simulink model "mfordmodel_v1"  (R2023a)
settings: Solver=ode45  StartTime=0.0  StopTime=10.0  RelTol=1e-3  EnableMultiTasking=on
undefined symbols (not defined in the file): ABV_RATIO_SW, AC_OFF_DLY, ACLOD, AUTO_TRNS_SW, BRAKE_DNDT_X, BZZRPM, BZZRPM_ALT, BZZTM, BZZTM_ALT, CMD_LITOFF, CMD_STABLE, CO_ST_ECT__A, COOL_BASE, DAS_BKDLY_A, DAS_CNT, DAS_CTDLY, DAS_LC_SW__A, DASCLP_5INH, DASCTL, DASMHYST, DASMPH, DEBYCP, DES_BASE, DPNEU_MUL, DSDRPM_DN_TC, DSDRPM_OFF, DSDRPM_UP_TC, EDF_DELAY, EDFHP, ETC_CL_TP, ETC_HP, GR_CM_CREEP, HCAM_ACT_CLP, HEDFHP, HEDFRPM, HICAM_PS, IAC_CAL_SW, IAC_ER_TM1, IAC_ER_TM2, IAC_ER_TM4, IAC_HI_LIM__A, IAC_ISFL_OBD, IAC_KAM_SW, IAC_LO_LIM__A, IAC_MON_TM, IAC_OT_REQ, IAC_RUN_TM, IAC_TP_OBD, IAC_TR_DAS, IAC_TST_DC, ID_DAS__A, ID_NOVS__A, IDVS_CH__A, IDVS_SL__A, IPSI_SW, IPSIDLY, IS_DRBASE__A, IS_DRBASE_A__A, IS_NUBASE__A, IS_NUBASE_A__A ... (+35)
libraries: simulink x2
(part 12 of 12)

== stateflow chart mfordmodel_v1/iac_v04_001_001/normal_mode/iscflg_module/idle_drive_rpm_controller/idle_drive_rpm_controller_ctl ==
  state idle_drive_rpm_init [parallel]
    settings: executionOrder=1
    idle_drive_rpm_init -> (junction 13) : trig
    (default) -> (junction 13) : trig
    (junction 13) -> (junction 14) : {
        | ml_init_sw = 2;
        | ml_idnerr_sw = 1;
        | do_idnerr_fil_calc;
        | do_idle_ppm_calc;
        | }
  state idle_drive_rpm_control [parallel]
    settings: executionOrder=2
    idle_drive_rpm_control -> (junction 15) : trig_idle_drive_rpm_controller
    (default) -> (junction 15) : trig_idle_drive_rpm_controller
    (junction 15) -> (junction 18) [order 2] : /* idle_drive_rpm_controller_initialisation() */
        | {
        | idle_drive_rpm_init.trig;
        | }
    (junction 15) -> (junction 16) [order 1] : [ ml_idrv_init_flg == 0 ]
        | {
        | ml_init_sw = 1;
        | do_idnerr_fil_calc;
        | }
    (junction 16) -> (junction 17) [order 2] : {
        | ml_idnerr_sw = 2;
        | }
    (junction 16) -> (junction 17) [order 1] : [ fabs(idnerr_fil) >= ID_DB_CAL ]
        | {
        | ml_idnerr_sw = 1;
        | }
    (junction 17) -> (junction 18) : {
        | do_idle_ppm_calc;
        | }
  data: ml_init_sw output uint8 size=1; ml_idrv_init_flg input boolean size=1; idnerr_fil input double size=1; ID_DB_CAL parameter double size=1; idnerr__A input double size=1; ml_idnerr_sw output int8 size=1
  events: trig local EITHER_EDGE_EVENT; trig_idle_drive_rpm_controller input FUNCTION_CALL_EVENT; do_idle_ppm_calc output FUNCTION_CALL_EVENT; do_idnerr_fil_calc output FUNCTION_CALL_EVENT

== stateflow chart mfordmodel_v1/iac_v04_001_001/normal_mode/activate_kam/activate_kam_ctl ==
  state isflag_update [parallel]
    settings: executionOrder=1
    isflag_update -> (junction 50) : trig   /* Determine which cell in 'isckam[]'
        |            will be used for learning: isflag =
        |            0 = No A/C request, neutral.
        |            1 = A/C request, neutral.
        |            2 = No A/C request, drive.
        |            3 = A/C request, drive.  */
    (default) -> (junction 50) : trig
    (junction 50) -> (junction 51) : {
        | islast = isflag;
        | }
    (junction 51) -> (junction 53) [order 1] : [ ac_ppm_rqst == 1 ]
        | {
        | isflag = 1;
        | }
    (junction 51) -> (junction 53) [order 2] : {
        | isflag = 0;
        | }
    (junction 53) -> (junction 55) [order 2]
    (junction 53) -> (junction 55) [order 1] : [ (dndsup == 0 )...
        |  || (AUTO_TRNS_SW == 0) ]
        | {
        | isflag = isflag + 2;
        | }
  state isckam_halt_logic [parallel]
    settings: executionOrder=2
    isckam_halt_logic -> (junction 48) : trig
    (default) -> (junction 48) : trig
    (junction 48) -> (junction 49) [order 1] : [ hicam < HICAM_LOW ]
    (junction 48) -> (junction 52) [order 2] : {
        |  hcamfg = 1;
        | }
    (junction 49) -> (junction 52) : [  ( is_source == IS_SOURCE_RPM_BASE_NEUTRAL_DRIVE)...
        |  || ( is_source == IS_SOURCE_HEATER_CORE_RPM)...
        |  || ( is_source == IS_SOURCE_AC_RPM) ]
        | {
        |  hcamfg = 0;
        | }
    (junction 52) -> (junction 54) [order 1] : [ (fabs(rpmerr_a) > RPMDED)...
        |  && ( iscflg == ISCFLG_RPM_CTRL_MODE) ]
        | {
        |  trig_iac_tmr_reset;
        | }
    (junction 52) -> (junction 54) [order 2] : {
        | trig_iac_tmr_update;
        | }
    (junction 54) -> (junction 60) [order 5] : {
        | isckam_hlt = 0;
        | }
    (junction 54) -> (junction 58) [order 1] : [   ( iac_kam_tmr < UPDISC )...
        |  || ( iscflg != ISCFLG_RPM_CTRL_MODE )...
        |  || ( hcamfg == 1 )...
        |  || ( isflag != islast )...
        |  || ( spk_source == 7 ) ]
    (junction 54) -> (junction 56) [order 4] : [  ( isflag == 1 )...
        |  || ( isflag == 3) ]
    (junction 54) -> (junction 58) [order 3] : [  ( PUR_ENA_SW >= 1 )...
        |   && ( pcomp_ena == 1 ) ]
    (junction 54) -> (junction 58) [order 2] : [  ( PRG_FLOW_SW == 1 )...
        |  && (flow_running == 1 ) ]
    (junction 56) -> (junction 58) : [ IAC_KAM_SW  == 1 ]
    (junction 58) -> (junction 60) : {
        | isckam_hlt = 1;
        | }
  state kam_qualification [parallel]
    settings: executionOrder=3
    kam_qualification -> (junction 57) : trig_isckam_qualification
    (default) -> (junction 57) : trig_isckam_qualification
    (junction 57) -> (junction 59) : {
        | do_kamsum_calc;
        | }
    (junction 59) -> (junction 62) [order 1] : [ ml_kamsum > 0.0 ]
        | {
        | do_isckam_clear;
        | }
    (junction 59) -> (junction 62) [order 2]
  state activate_kam [parallel]
    settings: executionOrder=4
    activate_kam -> (junction 61) : trig_activate_kam
    (default) -> (junction 61) : trig_activate_kam
    (junction 61) -> (junction 63) : {
        | isflag_update.trig;
        | isckam_halt_logic.trig;
        | /* BEGIN: isckam_update(); */
        | ipsibr_kam = ipsibr_fb;
        | }
    (junction 63) -> (junction 64) [order 2]
    (junction 63) -> (junction 70) [order 1] : [ ( kam_error == 1 )...
        |  || ( isckam[isflag] < PSIBRN )...
        |  || ( isckam[isflag] > PSIBRM ) ]
        | {
        | do_isckam_clear;
        | ibgpsi = 0;
        | }
    (junction 64) -> (junction 70) [order 1] : [ isckam_hlt == 1 ]
        | {
        | ibgpsi = 0;
        | }
    (junction 64) -> (junction 65) [order 2]
    (junction 65) -> (junction 67) [order 1] : [ ibgpsi >= UPDATM ]
        | {
        | ibgpsi = 0;
        | }
    (junction 65) -> (junction 66) [order 2]
    (junction 66) -> (junction 70) [order 1] : [ ibgpsi < IBGPSI_CLIP ]
        | {
        | ibgpsi++;
        | }
    (junction 66) -> (junction 70) [order 2]
    (junction 67) -> (junction 69) [order 1] : [ ipsibr_fb > 0.0 ]
        | {
        | ml_kam_inc_sw = 2;
        | }
    (junction 67) -> (junction 68) [order 2]
    (junction 68) -> (junction 69) [order 1] : [ ipsibr_fb < 0.0 ]
        | {
        | ml_kam_inc_sw = 1;
        | }
    (junction 68) -> (junction 69) [order 2] : {
        | ml_kam_inc_sw = 3;
        | }
    (junction 69) -> (junction 70) : {
        | ml_isflag_sw = isflag + 1;
        | do_isckam_calcs;
        | do_isckam_update_checksum;
        | }
    (junction 70) -> (junction 71) : {
        | do_update_pids;
        | }
  data: hcamfg output boolean size=1; is_source input uint8 size=1; rpmerr_a input double size=1; pcomp_ena input boolean size=1; flow_running input boolean size=1; iscflg input uint8 size=1; spk_source input uint8 size=1; dndsup input boolean size=1; ac_ppm_rqst input boolean size=1; isflag output uint8 size=1; ml_kam_inc_sw output uint8 size=1; PRG_FLOW_SW parameter boolean size=1; PUR_ENA_SW parameter boolean size=1; RPMDED parameter double size=1; UPDISC parameter double size=1; AUTO_TRNS_SW parameter boolean size=1; ml_isflag_sw output uint8 size=1; kam_error input boolean size=1; UPDATM parameter double size=1; PSIBRN parameter double size=1; PSIBRM parameter double size=1; ipsibr_fb input double size=1; hicam input double size=1; isckam input double size=4; IS_SOURCE_RPM_BASE_NEUTRAL_DRIVE constant uint8 size=1 =20; IS_SOURCE_HEATER_CORE_RPM constant uint8 size=1 =12; IS_SOURCE_AC_RPM constant uint8 size=1 =2; HICAM_LOW constant double size=1 =.003; islast output uint8 size=1; ibgpsi local uint8 size=1; ml_kamsum input double size=1; iac_kam_tmr input double size=1; IAC_KAM_SW parameter boolean size=1; ipsibr_kam output double size=1; IBGPSI_CLIP constant uint8 size=1 =255; ISCFLG_RPM_CTRL_MODE constant int8 size=1 =1; isckam_hlt local boolean size=1
  events: trig local EITHER_EDGE_EVENT; trig local EITHER_EDGE_EVENT; trig local EITHER_EDGE_EVENT; trig local EITHER_EDGE_EVENT; do_isckam_update_checksum output FUNCTION_CALL_EVENT; do_isckam_calcs output FUNCTION_CALL_EVENT; do_isckam_clear output FUNCTION_CALL_EVENT; do_update_pids output FUNCTION_CALL_EVENT; do_kamsum_calc output FUNCTION_CALL_EVENT; trig_iac_tmr_reset output FUNCTION_CALL_EVENT; trig_iac_tmr_update output FUNCTION_CALL_EVENT; trig_activate_kam input FUNCTION_CALL_EVENT; trig_isckam_qualification input FUNCTION_CALL_EVENT
